simulink model "modelo_simulink"  (R2015b)
settings: Solver=ode4  SolverMode=SingleTasking  StartTime=0.0  StopTime=T  RelTol=1e-3
values from neighbouring files (symbols this model uses):
  A1 = d*9.9    (= 59.4)    [AtorCritic4states.m]
  A2 = d*10    (= 60)    [AtorCritic4states.m]
  A3 = d*10    (= 60)    [AtorCritic4states.m]
  A4 = d*10    (= 60)    [AtorCritic4states.m]
  h1 = h1(end)    [AtorCritic4states.m]
  h2 = h2(end)    [AtorCritic4states.m]
  h3 = h3(end)    [AtorCritic4states.m]
  h4 = h4(end)    [AtorCritic4states.m]
  hmax = 1    [AtorCritic4states.m]
  k1 = 0    [AtorCritic4states.m]
  k12 = 9.06    [AtorCritic4states.m]
  k2 = 4.313    [AtorCritic4states.m]
  k23 = 11.89    [AtorCritic4states.m]
  k3 = 0    [AtorCritic4states.m]
  k34 = 10.09    [AtorCritic4states.m]
  k4 = 4.9667    [AtorCritic4states.m]
  T = 0.5    [AtorCritic4states.m]
settings Model: Creator=alvar  LastModifiedBy=alvar
settings DataIOCC: LimitDataPoints=off
settings DebuggingCC: AllowSymbolicDim=on  SFUnexpectedBacktrackingDiag=error  SFNoUnconditionalDefaultTransitionDiag=error
settings ModelReferenceCC: PropagateSignalLabelsOutOfModel=on
settings GRTTargetCC: TargetLangStandard=C99 (ISO)
settings ConfigComp: CovMetricSettings=dwe  CovHtmlReporting=off  CovSaveCumulativeToWorkspaceVar=off  CovSaveSingleToWorkspaceVar=off  CovModelRefEnable=Off  CovExternalEMLEnable=on

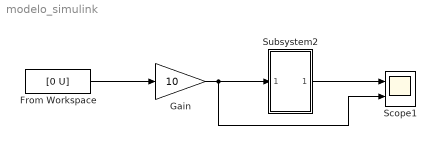
== system modelo_simulink ==
  From Workspace : FromWorkspace  VariableName=[0 U]  SampleTime=T
  Gain : Gain  Gain=10
  Scope1 : Scope  NumInputPorts=2
  Subsystem2 : Subsystem
  wires:
  Subsystem2/1(Out1) -> Scope1/1
  Gain/1 -> Scope1/2, Subsystem2/1(In1)
  From Workspace/1 -> Gain/1

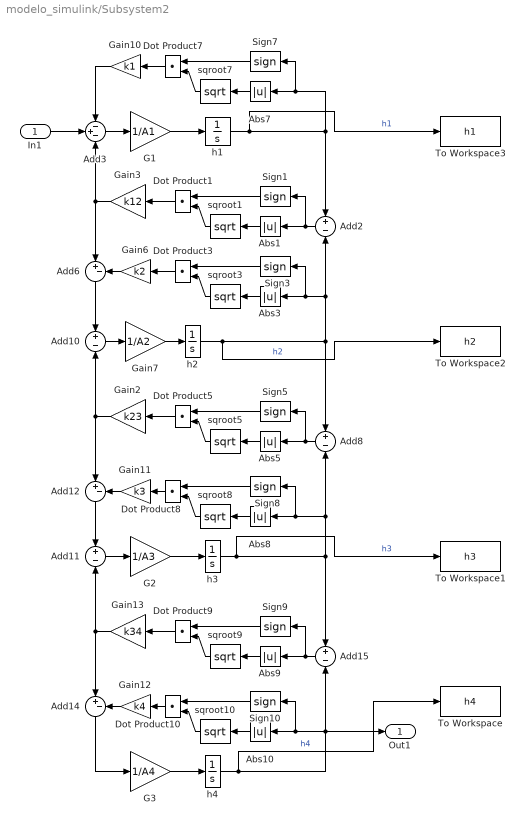
== system modelo_simulink/Subsystem2 ==
  In1 : Inport
  Abs{1,3,5,7..10} (7 alike) : Abs
  Add{2,8,10..11,15} (5 alike) : Sum  Inputs=+-
  Add12 : Sum  Inputs=|+-
  Add14 : Sum  Inputs=|+-
  Add3 : Sum  Inputs=-+-
  Add6 : Sum  Inputs=|+-
  Dot Product{1,3,5,7..10} (7 alike) : DotProduct  InputSameDT=on  OutDataTypeStr=Inherit: Inherit via internal rule
  G1 : Gain  Gain=1/A1
  G2 : Gain  Gain=1/A3
  G3 : Gain  Gain=1/A4
  Gain10 : Gain  Gain=k1
  Gain11 : Gain  Gain=k3
  Gain12 : Gain  Gain=k4
  Gain13 : Gain  Gain=k34
  Gain2 : Gain  Gain=k23
  Gain3 : Gain  Gain=k12
  Gain6 : Gain  Gain=k2
  Gain7 : Gain  Gain=1/A2
  Sign{1,3,5,7..10} (7 alike) : Signum
  To Workspace : ToWorkspace  VariableName=h4  SampleTime=T
  To Workspace1 : ToWorkspace  VariableName=h3  SampleTime=T
  To Workspace2 : ToWorkspace  VariableName=h2  SampleTime=T
  To Workspace3 : ToWorkspace  VariableName=h1  SampleTime=T
  h1 : Integrator  InitialCondition=h1  LimitOutput=on  UpperSaturationLimit=hmax  LowerSaturationLimit=0
  h2 : Integrator  InitialCondition=h2  LimitOutput=on  UpperSaturationLimit=hmax  LowerSaturationLimit=0
  h3 : Integrator  InitialCondition=h3  LimitOutput=on  UpperSaturationLimit=hmax  LowerSaturationLimit=0
  h4 : Integrator  InitialCondition=h4  LimitOutput=on  UpperSaturationLimit=hmax  LowerSaturationLimit=0
  sqroot{1,3,5,7..10} (7 alike) : Math  Operator=sqrt  SaturateOnIntegerOverflow=on
  Out1 : Outport
  wires:
  Add2/1 -> Abs1/1, Sign1/1
  Abs1/1 -> sqroot1/1
  Sign1/1 -> Dot Product1/1
  sqroot1/1 -> Dot Product1/2
  Dot Product1/1 -> Gain3/1
  Add3/1 -> G1/1
  Gain3/1 -> Add6/1, Add3/3
  G1/1 -> h1/1
  Abs3/1 -> sqroot3/1
  Sign3/1 -> Dot Product3/1
  sqroot3/1 -> Dot Product3/2
  Dot Product3/1 -> Gain6/1
  Gain7/1 -> h2/1
  Gain6/1 -> Add6/2
  Add8/1 -> Abs5/1, Sign5/1
  Abs5/1 -> sqroot5/1
  Sign5/1 -> Dot Product5/1
  sqroot5/1 -> Dot Product5/2
  Dot Product5/1 -> Gain2/1
  Gain2/1 -> Add10/2, Add12/1
  Abs7/1 -> sqroot7/1
  Sign7/1 -> Dot Product7/1
  sqroot7/1 -> Dot Product7/2
  Dot Product7/1 -> Gain10/1
  Gain10/1 -> Add3/1
  Add6/1 -> Add10/1
  Add10/1 -> Gain7/1
  Add11/1 -> G2/1
  G2/1 -> h3/1
  Abs8/1 -> sqroot8/1
  Sign8/1 -> Dot Product8/1
  sqroot8/1 -> Dot Product8/2
  Dot Product8/1 -> Gain11/1
  Gain11/1 -> Add12/2
  Add12/1 -> Add11/1
  Add15/1 -> Abs9/1, Sign9/1
  Abs9/1 -> sqroot9/1
  Sign9/1 -> Dot Product9/1
  sqroot9/1 -> Dot Product9/2
  Dot Product9/1 -> Gain13/1
  Gain13/1 -> Add14/1, Add11/2
  Add14/1 -> G3/1
  G3/1 -> h4/1
  Abs10/1 -> sqroot10/1
  Sign10/1 -> Dot Product10/1
  sqroot10/1 -> Dot Product10/2
  Dot Product10/1 -> Gain12/1
  Gain12/1 -> Add14/2
  h4/1 -> Out1/1, Add15/2, Abs10/1, Sign10/1, To Workspace/1  "h4"
  h3/1 -> Add15/1, Abs8/1, Sign8/1, Add8/2, To Workspace1/1  "h3"
  h2/1 -> Add2/2, Abs3/1, Sign3/1, Add8/1, To Workspace2/1  "h2"
  h1/1 -> Add2/1, Abs7/1, Sign7/1, To Workspace3/1  "h1"
  In1/1 -> Add3/2
